simulink model "M010_refor_control_SOFC"  (R2021a)
settings: Solver=ode23tb  StartTime=0.0  StopTime=Tf  RelTol=1e-3
values from neighbouring files (symbols this model uses):
  Diesel = Diesel*rho_diesel    (= 9.22132410008e-05)    [M010_init_refor_SOFC.m]
  MM_vec = struct2array(MM)'    [M010_init_refor_SOFC.m]
settings Model: Creator=djoroya  LastModifiedBy=djoroya

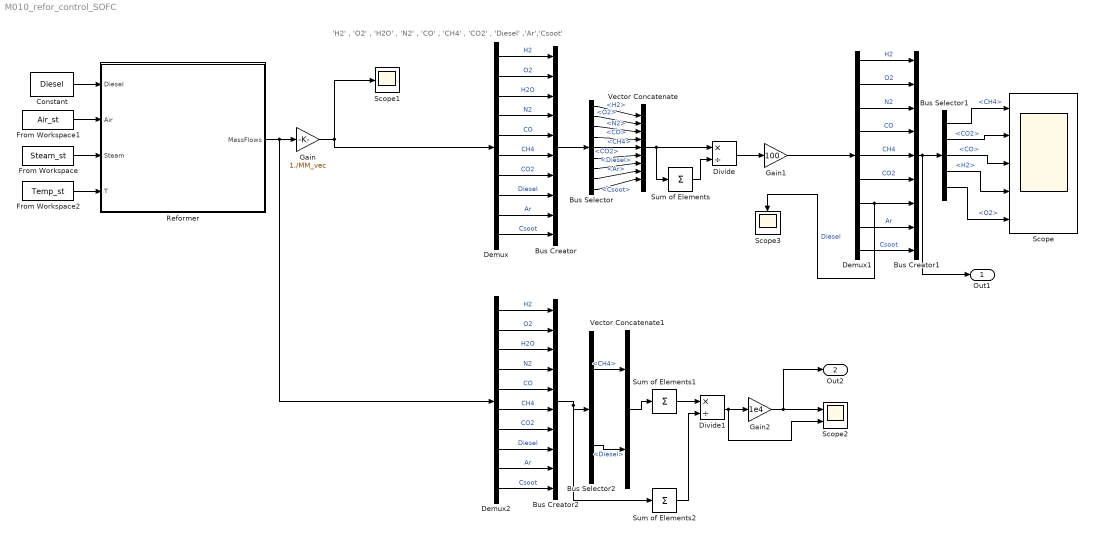
== system M010_refor_control_SOFC ==
  note: 'H2' , 'O2' , 'H2O' , 'N2' , 'CO' , 'CH4' , 'CO2' , 'Diesel' ,'Ar','Csoot'
  Bus Creator : BusCreator  Inputs=10
  Bus Creator1 : BusCreator  Inputs=9
  Bus Creator2 : BusCreator  Inputs=10
  Bus Selector : BusSelector  OutputSignals=H2,O2,N2,CO,CH4,CO2,Diesel,Ar,Csoot
  Bus Selector1 : BusSelector  OutputSignals=CH4,CO2,CO,H2,O2
  Bus Selector2 : BusSelector  OutputSignals=CH4,Diesel
  Constant : Constant  Value=Diesel
  Demux : Demux  Outputs=10
  Demux1 : Demux  Outputs=9
  Demux2 : Demux  Outputs=10
  Divide : Product  Inputs=*/
  Divide1 : Product  Inputs=*/
  From Workspace : FromWorkspace  VariableName=Steam_st
  From Workspace1 : FromWorkspace  VariableName=Air_st
  From Workspace2 : FromWorkspace  VariableName=Temp_st
  Gain : Gain  Gain=1./MM_vec
  Gain1 : Gain  Gain=100
  Gain2 : Gain  Gain=1e4
  "Reformer " : Subsystem
  Scope : Scope  NumInputPorts=5
  Scope1 : Scope
  Scope2 : Scope  NumInputPorts=2
  Scope3 : Scope
  Sum of Elements : Sum  Inputs=+
  Sum of Elements1 : Sum  Inputs=+
  Sum of Elements2 : Sum  Inputs=+
  Vector Concatenate : Concatenate  NumInputs=9
  Vector Concatenate1 : Concatenate
  Out1 : Outport
  Out2 : Outport  Port=2
  wires:
  Constant/1 -> "Reformer "/1(Diesel)
  From Workspace/1 -> "Reformer "/3(Steam)
  From Workspace1/1 -> "Reformer "/2(Air)
  From Workspace2/1 -> "Reformer "/4(T)
  Demux/1 -> Bus Creator/1  "H2"
  Demux/2 -> Bus Creator/2  "O2"
  Demux/3 -> Bus Creator/3  "H2O"
  Demux/4 -> Bus Creator/4  "N2"
  Demux/5 -> Bus Creator/5  "CO"
  Demux/6 -> Bus Creator/6  "CH4"
  Demux/7 -> Bus Creator/7  "CO2"
  Demux/8 -> Bus Creator/8  "Diesel"
  Demux/9 -> Bus Creator/9  "Ar"
  Demux/10 -> Bus Creator/10  "Csoot"
  Bus Creator/1 -> Bus Selector/1
  "Reformer "/1(MassFlows) -> Demux2/1, Gain/1
  Gain/1 -> Demux/1, Scope1/1
  Bus Selector/9 -> Vector Concatenate/9  "<Csoot>"
  Bus Selector/8 -> Vector Concatenate/8  "<Ar>"
  Bus Selector/7 -> Vector Concatenate/7  "<Diesel>"
  Bus Selector/6 -> Vector Concatenate/6  "<CO2>"
  Bus Selector/5 -> Vector Concatenate/5  "<CH4>"
  Bus Selector/4 -> Vector Concatenate/4  "<CO>"
  Bus Selector/3 -> Vector Concatenate/3  "<N2>"
  Bus Selector/1 -> Vector Concatenate/1  "<H2>"
  Bus Selector/2 -> Vector Concatenate/2  "<O2>"
  Vector Concatenate/1 -> Divide/1, Sum of Elements/1
  Sum of Elements/1 -> Divide/2
  Demux1/8 -> Bus Creator1/8  "Ar"
  Demux1/4 -> Bus Creator1/4  "CO"
  Demux1/6 -> Bus Creator1/6  "CO2"
  Demux1/3 -> Bus Creator1/3  "N2"
  Demux1/5 -> Bus Creator1/5  "CH4"
  Demux1/7 -> Scope3/1, Bus Creator1/7  "Diesel"
  Demux1/9 -> Bus Creator1/9  "Csoot"
  Demux1/1 -> Bus Creator1/1  "H2"
  Demux1/2 -> Bus Creator1/2  "O2"
  Bus Creator1/1 -> Bus Selector1/1, Out1/1
  Divide/1 -> Gain1/1
  Gain1/1 -> Demux1/1
  Bus Selector1/1 -> Scope/1  "<CH4>"
  Bus Selector1/2 -> Scope/2  "<CO2>"
  Bus Selector1/3 -> Scope/3  "<CO>"
  Bus Selector1/4 -> Scope/4  "<H2>"
  Bus Selector1/5 -> Scope/5  "<O2>"
  Bus Creator2/1 -> Sum of Elements2/1, Bus Selector2/1
  Demux2/5 -> Bus Creator2/5  "CO"
  Demux2/2 -> Bus Creator2/2  "O2"
  Demux2/4 -> Bus Creator2/4  "N2"
  Demux2/3 -> Bus Creator2/3  "H2O"
  Demux2/9 -> Bus Creator2/9  "Ar"
  Demux2/6 -> Bus Creator2/6  "CH4"
  Demux2/10 -> Bus Creator2/10  "Csoot"
  Demux2/7 -> Bus Creator2/7  "CO2"
  Demux2/8 -> Bus Creator2/8  "Diesel"
  Demux2/1 -> Bus Creator2/1  "H2"
  Bus Selector2/1 -> Vector Concatenate1/1  "<CH4>"
  Bus Selector2/2 -> Vector Concatenate1/2  "<Diesel>"
  Vector Concatenate1/1 -> Sum of Elements1/1
  Sum of Elements1/1 -> Divide1/1
  Sum of Elements2/1 -> Divide1/2
  Divide1/1 -> Scope2/2, Gain2/1
  Gain2/1 -> Out2/1, Scope2/1

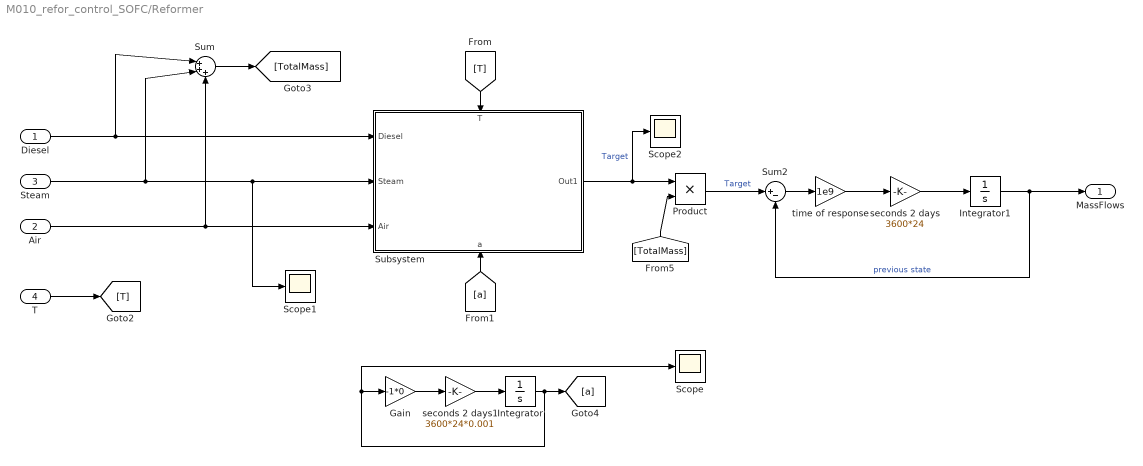
== system M010_refor_control_SOFC/Reformer  ==
  Diesel : Inport
  Air : Inport  Port=2
  Steam : Inport  Port=3
  T : Inport  Port=4
  Gain : Gain  Gain=-1*0
  Integrator : Integrator  InitialCondition=1
  Integrator1 : Integrator  InitialCondition=1e-6
  Product : Product
  Scope : Scope
  Scope1 : Scope
  Scope2 : Scope
  Subsystem : Subsystem
      settings: PortSchema="{\"entries\":[{\"content\":{\"sides\":[{\"content\":{\"connectorIds\":[\"In1\",\"In2\",\"In3\"]},\"type\":\"ConnectorPlacement.EquallySpacedRectSide\",\"uuid\":\"0dada652-6957-4c3e-8e48-73ee360a3bab\"},{\"content\":{\"connectorIds\":[\"Out1\"],\"side\":\"RIGHT\"},\"type\":\"ConnectorPlacement.EquallySpacedRectSide\",\"uuid\":\"81208621-951c-43f9-b655-3502a16ce57a\"},{\"content\":{\"connectorIds\":[\"In4\"],\"side\":\"TOP\"},\"type\":\"ConnectorPlacement.EquallySpacedRectSide\",\"uuid\":\"1012e2be-7d0b-44a9-9a40-bc453950010e\"},{\"content\":{\"connectorIds\":[\"In5\"],\"side\":\"BOTTOM\"},\"type\":\"ConnectorPlacement.EquallySpacedRectSide\",\"uuid\":\"aaef83a2-abb7-4780-82b5-9abad57d39ad\"}]},\"type\":\"ConnectorPlacement.EquallySpacedConnector\",\"uuid\":\"1143871f-aacc-4fa7-a444-9910d5016eff\"}],\"packageUris\":[\"http://schema.mathworks.com/mf0/Connector/R2020b\"],\"version\":\"1.0\"}"
  Sum : Sum  Inputs=|+++
  Sum2 : Sum  Inputs=|+-
  seconds 2 days : Gain  Gain=3600*24
  seconds 2 days1 : Gain  Gain=3600*24*0.001
  time of response : Gain  Gain=1e9
  MassFlows : Outport
  wires:
  T/1 -> [T]
  Sum/1 -> [TotalMass]
  [TotalMass] -> Product/2
  Diesel/1 -> Sum/1, Subsystem/1(Diesel)
  seconds 2 days1/1 -> Integrator/1
  Gain/1 -> seconds 2 days1/1
  [a] -> Subsystem/5(a)
  [T] -> Subsystem/4(T)
  time of response/1 -> seconds 2 days/1
  Sum2/1 -> time of response/1
  Product/1 -> Sum2/1  "Target"
  seconds 2 days/1 -> Integrator1/1
  Integrator1/1 -> MassFlows/1, Sum2/2  "previous state"
  Subsystem/1(Out1) -> Scope2/1, Product/1  "Target"
  Steam/1 -> Sum/2, Scope1/1, Subsystem/2(Steam)
  Air/1 -> Sum/3, Subsystem/3(Air)
  Integrator/1 -> Scope/1, Gain/1, [a]

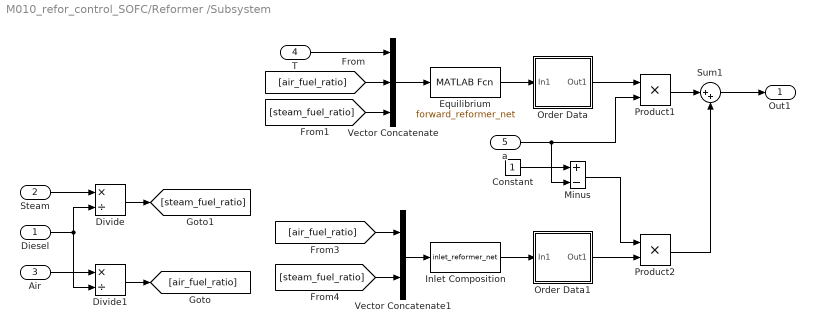
== system M010_refor_control_SOFC/Reformer /Subsystem ==
  Diesel : Inport
  Steam : Inport  Port=2
  Air : Inport  Port=3
  T : Inport  Port=4
  a : Inport  Port=5
  Constant : Constant
  Divide : Product  Inputs=*/
  Divide1 : Product  Inputs=*/
  Equilibrium : MATLABFcn  MATLABFcn=forward_reformer_net  OutputDimensions=8  OutputSignalType=real  Output1D=off
  Inlet Composition : MATLABFcn  MATLABFcn=inlet_reformer_net  OutputDimensions=6  OutputSignalType=real  Output1D=off
  Minus : Sum  Inputs=+-
  Order Data : Subsystem
  Order Data1 : Subsystem
  Product1 : Product
  Product2 : Product
  Sum1 : Sum  Inputs=|++
  Vector Concatenate : Concatenate  NumInputs=3
  Vector Concatenate1 : Concatenate
  Out1 : Outport
  wires:
  a/1 -> Product1/2, Minus/2
  [steam_fuel_ratio] -> Vector Concatenate/3
  Product1/1 -> Sum1/1
  T/1 -> Vector Concatenate/1
  [air_fuel_ratio] -> Vector Concatenate1/1
  Vector Concatenate/1 -> Equilibrium/1
  Product2/1 -> Sum1/2
  [steam_fuel_ratio] -> Vector Concatenate1/2
  Order Data1/1(Out1) -> Product2/2
  Minus/1 -> Product2/1
  Inlet Composition/1 -> Order Data1/1(In1)
  Order Data/1(Out1) -> Product1/1
  Vector Concatenate1/1 -> Inlet Composition/1
  [air_fuel_ratio] -> Vector Concatenate/2
  Equilibrium/1 -> Order Data/1(In1)
  Constant/1 -> Minus/1
  Sum1/1 -> Out1/1
  Steam/1 -> Divide/1
  Diesel/1 -> Divide1/2, Divide/2
  Air/1 -> Divide1/1
  Divide/1 -> [steam_fuel_ratio]
  Divide1/1 -> [air_fuel_ratio]

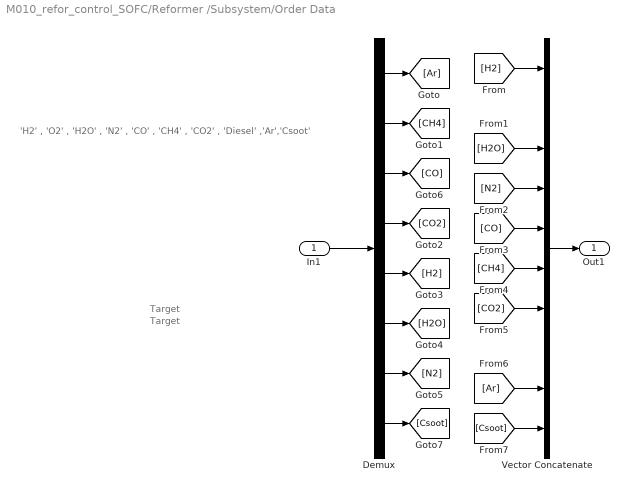
== system M010_refor_control_SOFC/Reformer /Subsystem/Order Data ==
  note: Target
  note: Target
  note: 'H2' , 'O2' , 'H2O' , 'N2' , 'CO' , 'CH4' , 'CO2' , 'Diesel' ,'Ar','Csoot'
  In1 : Inport
  Demux : Demux  Outputs=8
  Vector Concatenate : Concatenate  NumInputs=10
  Out1 : Outport
  wires:
  In1/1 -> Demux/1
  Demux/1 -> [Ar]
  Demux/2 -> [CH4]
  Demux/3 -> [CO]
  Demux/4 -> [CO2]
  Demux/5 -> [H2]
  Demux/6 -> [H2O]
  Demux/7 -> [N2]
  Demux/8 -> [Csoot]
  [H2] -> Vector Concatenate/1
  [H2O] -> Vector Concatenate/3
  [N2] -> Vector Concatenate/4
  [CO] -> Vector Concatenate/5
  [CH4] -> Vector Concatenate/6
  [CO2] -> Vector Concatenate/7
  [Ar] -> Vector Concatenate/9
  [Csoot] -> Vector Concatenate/10
  Vector Concatenate/1 -> Out1/1

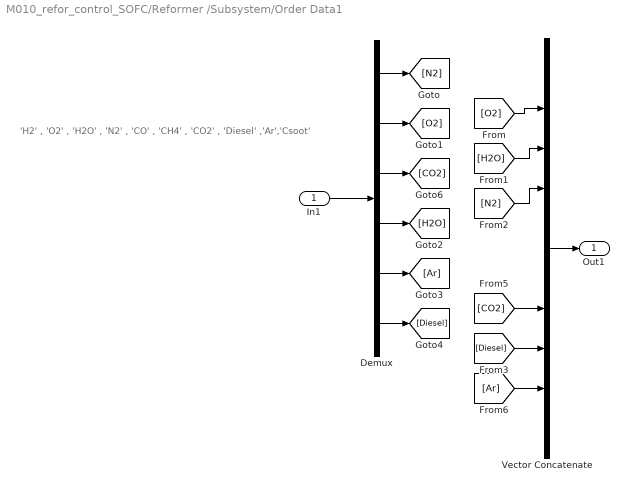
== system M010_refor_control_SOFC/Reformer /Subsystem/Order Data1 ==
  note: 'H2' , 'O2' , 'H2O' , 'N2' , 'CO' , 'CH4' , 'CO2' , 'Diesel' ,'Ar','Csoot'
  In1 : Inport
  Demux : Demux  Outputs=6
  Vector Concatenate : Concatenate  NumInputs=10
  Out1 : Outport
  wires:
  In1/1 -> Demux/1
  Demux/1 -> [N2]
  Demux/2 -> [O2]
  Demux/3 -> [CO2]
  Demux/4 -> [H2O]
  Demux/5 -> [Ar]
  Demux/6 -> [Diesel]
  [H2O] -> Vector Concatenate/3
  [N2] -> Vector Concatenate/4
  [CO2] -> Vector Concatenate/7
  [Ar] -> Vector Concatenate/9
  Vector Concatenate/1 -> Out1/1
  [O2] -> Vector Concatenate/2
  [Diesel] -> Vector Concatenate/8
